simulink model "pra_tirar_print"  (R2016a)
settings: Solver=ode14x  StartTime=0.0  StopTime=30  FixedStep=0.001  RelTol=1e-3
InitFcn:
  | clear all;
  | Kpx = 10;
  | Kix = 25;
  | Kpy = 10;
  | Kiy = 25;
  | Kvphi = 3;
  | Kpphi = 2.25;
  | 
  | Kem = 0.0059;
  | Kti = 0.0059;
  | Vd = 5.4;
  | R = 1.71;
  | r = 0.072;
  | eta = 0.83;
  | N = 19;
  | 
  | Jw = 8.1e-4;
  | 
  | mi = 0.25;
  | b = .1;
  | 
  | Ts = 0.01;
  | 
  | 
  | alpha1 = 0;
  | alpha2 = 120*pi/180;
  | alpha3 = 240*pi/180;
  | g = 9.8;
  | vs = 6e-10;
  | M = 1.83;
  | l1 = 0.09;
  | l2 = 0.09;
  | l3 = 0.09;
  | r1 = 0.072;
  | r2 = 0.072;
  | r3 = 0.072;
  | kt = 0.0059;
  | kem = 0.0059;
  | N = 19;
  | L = 0.00011;
  | R = 1.71;
  | Jm1 = 3.88e-7;
  | Jm2 = 3.88e-7;
  | Jm3 = 3.88e-7;
  | J1 = 8.1e-4;
  | J2 = 8.1e-4;
  | J3 = 8.1e-4;
  | J = 2.125;
  | eta = 0.83;
  | freq = 1000; % varia entre 2.5kHz e 5Mhz
  | mic = 0.25;
  | mis = 0.25;
  | sigma0 = 100;
  | sigma1 = 0.1;
  | sigma2 = 0.1;
  | 
  | mi = 0.25;
  | b = .1;
  | 
  | kctr = kt*5.4*eta*N/(R*r1)
libraries: simulink x1
settings Model: Creator=Pichau  LastModifiedBy=Pichau

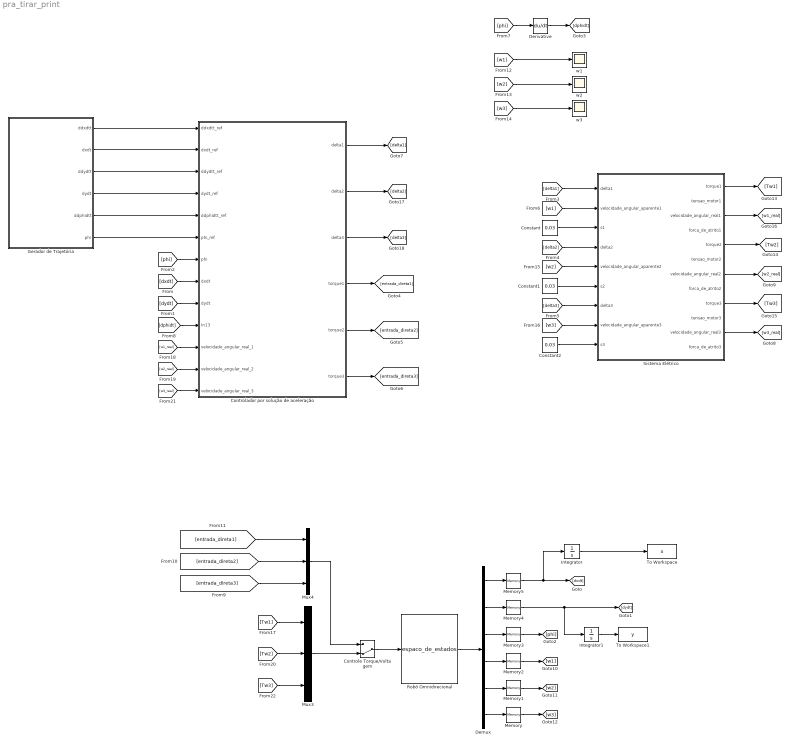
== system pra_tirar_print ==
  Constant : Constant  Value=0.03
  Constant1 : Constant  Value=0.03
  Constant2 : Constant  Value=0.03
  Controlador por solução de aceleração : Subsystem
  Controle Torque/Voltagem : ManualSwitch  CurrentSetting=0
  Demux : Demux  Outputs=6
  Derivative : Derivative
  Gerador de Trajetória : Subsystem
  Integrator : Integrator  InitialCondition=0.3
  Integrator1 : Integrator
  Memory{,1..2,4..5} (5 alike) : Memory
  Memory3 : Memory  X0=pi/2
  Mux3 : Mux  Inputs=3
  Mux4 : Mux  Inputs=3
  Robô Omnidirecional : S-Function  FunctionName=espaco_de_estados  Parameters=r,m,Jw,J,L  SFunctionDeploymentMode=off  EnableBusSupport=off  mask{r=0.072, m=1.71, Jw=8.1e-4, J=2.125, L=0.09}
      mask prompts: r "r (m)"; m "m (Kg)"; Jw "Jw (Kg*m^2)"; J "J (Kg*m^2)"; L "L (m)"
      mask Display: image(imread('Robot_omnidirectional_drive.png'));
  Sistema Elétrico : Subsystem
  To Workspace : ToWorkspace  VariableName=x  SaveFormat=Timeseries  SampleTime=-1
  To Workspace1 : ToWorkspace  VariableName=y  SaveFormat=Timeseries  SampleTime=-1
  w1 : Scope
  w2 : Scope
  w3 : Scope
  wires:
  Robô Omnidirecional/1 -> Demux/1
  Integrator1/1 -> To Workspace1/1
  Integrator/1 -> To Workspace/1
  Derivative/1 -> [dphidt]
  Mux3/1 -> Controle Torque/Voltagem/2
  Controle Torque/Voltagem/1 -> Robô Omnidirecional/1
  [w3] -> w3/1
  [w2] -> w2/1
  [w1] -> w1/1
  Demux/1 -> Memory5/1
  Demux/2 -> Memory4/1
  [phi] -> Derivative/1
  Demux/4 -> Memory2/1
  Demux/5 -> Memory1/1
  Demux/6 -> Memory/1
  Mux4/1 -> Controle Torque/Voltagem/1
  Memory/1 -> [w3]
  Memory1/1 -> [w2]
  Memory2/1 -> [w1]
  Memory4/1 -> [dydt], Integrator1/1
  Memory5/1 -> Integrator/1, [dxdt]
  Memory3/1 -> [phi]
  [entrada_direta3] -> Mux4/3
  [entrada_direta2] -> Mux4/2
  [entrada_direta1] -> Mux4/1
  Demux/3 -> Memory3/1
  Sistema Elétrico/5(torque2) -> [Tw2]
  Sistema Elétrico/9(torque3) -> [Tw3]
  Sistema Elétrico/1(torque1) -> [Tw1]
  [w1] -> Sistema Elétrico/2(velocidade_angular_aparente1)
  [delta2] -> Sistema Elétrico/4(delta2)
  [w2] -> Sistema Elétrico/5(velocidade_angular_aparente2)
  [delta3] -> Sistema Elétrico/7(delta3)
  [w3] -> Sistema Elétrico/8(velocidade_angular_aparente3)
  Sistema Elétrico/3(velocidade_angular_real1) -> [w1_real]
  Sistema Elétrico/7(velocidade_angular_real2) -> [w2_real]
  Sistema Elétrico/11(velocidade_angular_real3) -> [w3_real]
  [Tw1] -> Mux3/1
  [Tw2] -> Mux3/2
  [Tw3] -> Mux3/3
  Gerador de Trajetória/1(ddxdtt) -> Controlador por solução de aceleração/1(ddxdtt_ref)
  Gerador de Trajetória/2(dxdt) -> Controlador por solução de aceleração/2(dxdt_ref)
  Gerador de Trajetória/3(ddydtt) -> Controlador por solução de aceleração/3(ddydtt_ref)
  Gerador de Trajetória/4(dydt) -> Controlador por solução de aceleração/4(dydt_ref)
  Gerador de Trajetória/5("ddphidtt ") -> Controlador por solução de aceleração/5(ddphidtt_ref)
  Gerador de Trajetória/6(phi) -> Controlador por solução de aceleração/6(phi_ref)
  [phi] -> Controlador por solução de aceleração/7(phi)
  [dxdt] -> Controlador por solução de aceleração/8(dxdt)
  [dydt] -> Controlador por solução de aceleração/9(dydt)
  [dphidt] -> Controlador por solução de aceleração/10(In13)
  [w2_real] -> Controlador por solução de aceleração/12(velocidade_angular_real_2)
  [w3_real] -> Controlador por solução de aceleração/13(velocidade_angular_real_3)
  [w1_real] -> Controlador por solução de aceleração/11(velocidade_angular_real_1)
  Controlador por solução de aceleração/5(torque2) -> [entrada_direta2]
  Controlador por solução de aceleração/6(torque3) -> [entrada_direta3]
  Controlador por solução de aceleração/4(torque1) -> [entrada_direta1]
  Controlador por solução de aceleração/1(delta1) -> [delta1]
  Controlador por solução de aceleração/2(delta2) -> [delta2]
  Controlador por solução de aceleração/3(delta3) -> [delta3]
  [delta1] -> Sistema Elétrico/1(delta1)
  Constant/1 -> Sistema Elétrico/3(s1)
  Constant1/1 -> Sistema Elétrico/6(s2)
  Constant2/1 -> Sistema Elétrico/9(s3)

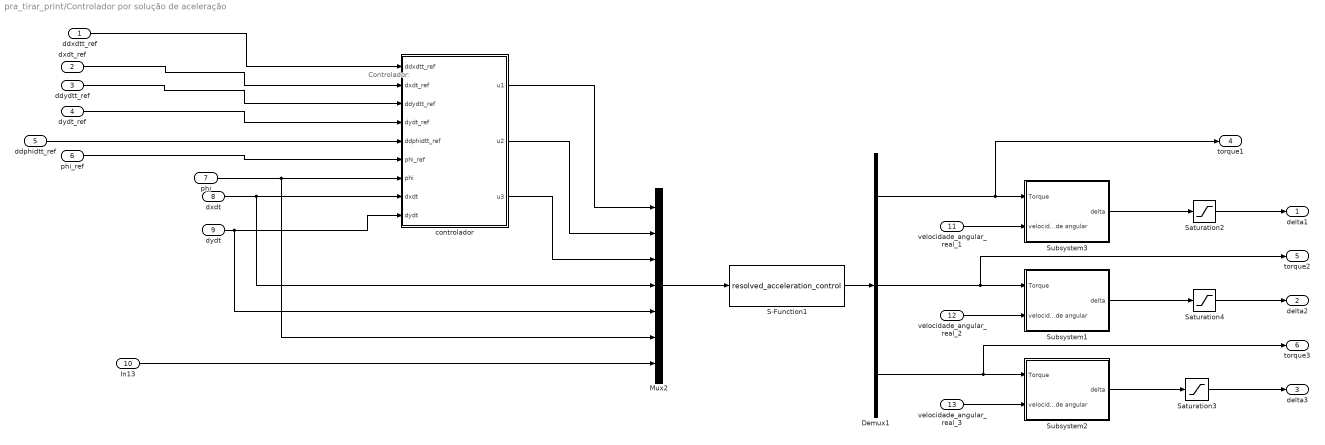
== system pra_tirar_print/Controlador por solução de aceleração ==
  note: Controlador:
  ddxdtt_ref : Inport
  dxdt_ref : Inport  Port=2
  ddydtt_ref : Inport  Port=3
  dydt_ref : Inport  Port=4
  ddphidtt_ref : Inport  Port=5
  phi_ref : Inport  Port=6
  phi : Inport  Port=7
  dxdt : Inport  Port=8
  dydt : Inport  Port=9
  In13 : Inport  Port=10
  velocidade_angular_real_1 : Inport  Port=11
  velocidade_angular_real_2 : Inport  Port=12
  velocidade_angular_real_3 : Inport  Port=13
  Demux1 : Demux  Outputs=3
  Mux2 : Mux  Inputs=7
  S-Function1 : S-Function  FunctionName=resolved_acceleration_control  Parameters=r,L,m,J,Jw  SFunctionDeploymentMode=off  EnableBusSupport=off  mask{r=0.072, L=0.09, m=1.71, J=2.125, Jw=8.1e-4}
  Saturation2 : Saturate  UpperLimit=1  LowerLimit=-1
  Saturation3 : Saturate  UpperLimit=1  LowerLimit=-1
  Saturation4 : Saturate  UpperLimit=1  LowerLimit=-1
  Subsystem1 : Subsystem
  Subsystem2 : Subsystem
  Subsystem3 : Subsystem
  controlador : Subsystem
  delta1 : Outport
  delta2 : Outport  Port=2
  delta3 : Outport  Port=3
  torque1 : Outport  Port=4
  torque2 : Outport  Port=5
  torque3 : Outport  Port=6
  wires:
  controlador/1(u1) -> Mux2/1
  controlador/3(u3) -> Mux2/3
  controlador/2(u2) -> Mux2/2
  Demux1/3 -> torque3/1, Subsystem2/1(Torque)
  ddxdtt_ref/1 -> controlador/1(ddxdtt_ref)
  dydt_ref/1 -> controlador/4(dydt_ref)
  ddydtt_ref/1 -> controlador/3(ddydtt_ref)
  dxdt_ref/1 -> controlador/2(dxdt_ref)
  phi/1 -> Mux2/6, controlador/7(phi)
  S-Function1/1 -> Demux1/1
  ddphidtt_ref/1 -> controlador/5(ddphidtt_ref)
  dxdt/1 -> Mux2/4, controlador/8(dxdt)
  dydt/1 -> Mux2/5, controlador/9(dydt)
  phi_ref/1 -> controlador/6(phi_ref)
  Mux2/1 -> S-Function1/1
  velocidade_angular_real_3/1 -> Subsystem2/2(velocidade angular)
  Subsystem2/1(delta) -> Saturation3/1
  velocidade_angular_real_1/1 -> Subsystem3/2(velocidade angular)
  Subsystem3/1(delta) -> Saturation2/1
  velocidade_angular_real_2/1 -> Subsystem1/2(velocidade angular)
  Demux1/1 -> torque1/1, Subsystem3/1(Torque)
  Subsystem1/1(delta) -> Saturation4/1
  In13/1 -> Mux2/7
  Saturation2/1 -> delta1/1
  Demux1/2 -> torque2/1, Subsystem1/1(Torque)
  Saturation3/1 -> delta3/1
  Saturation4/1 -> delta2/1

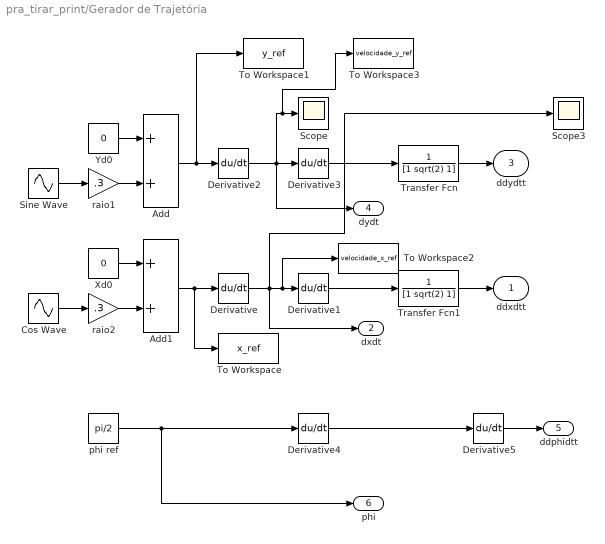
== system pra_tirar_print/Gerador de Trajetória ==
  Add : Sum
  Add1 : Sum
  Cos Wave : Sin  Frequency=0.3  Phase=pi/2  SampleTime=0
  Derivative{,1..5} (6 alike) : Derivative
  Scope : Scope
  Scope3 : Scope
  Sine Wave : Sin  Frequency=0.3  SampleTime=0
  To Workspace : ToWorkspace  VariableName=x_ref  SaveFormat=Timeseries  SampleTime=-1
  To Workspace1 : ToWorkspace  VariableName=y_ref  SaveFormat=Timeseries  SampleTime=-1
  To Workspace2 : ToWorkspace  VariableName=velocidade_x_ref  SaveFormat=Timeseries  SampleTime=-1
  To Workspace3 : ToWorkspace  VariableName=velocidade_y_ref  SaveFormat=Timeseries  SampleTime=-1
  Transfer Fcn : TransferFcn  Denominator=[1 sqrt(2) 1]
  Transfer Fcn1 : TransferFcn  Denominator=[1 sqrt(2) 1]
  Xd0 : Constant  Value=0
  Yd0 : Constant  Value=0
  phi ref : Constant  Value=pi/2
  raio1 : Gain  Gain=.3
  raio2 : Gain  Gain=.3
  ddxdtt : Outport
  dxdt : Outport  Port=2
  ddydtt : Outport  Port=3
  dydt : Outport  Port=4
  "ddphidtt " : Outport  Port=5
  phi : Outport  Port=6
  wires:
  Transfer Fcn1/1 -> ddxdtt/1
  Transfer Fcn/1 -> ddydtt/1
  Derivative1/1 -> Transfer Fcn1/1
  Derivative3/1 -> Transfer Fcn/1
  Derivative2/1 -> Derivative3/1, To Workspace3/1, Scope/1, dydt/1
  Derivative/1 -> Scope3/1, To Workspace2/1, Derivative1/1, dxdt/1
  Sine Wave/1 -> raio1/1
  raio1/1 -> Add/2
  Add/1 -> To Workspace1/1, Derivative2/1
  Add1/1 -> To Workspace/1, Derivative/1
  raio2/1 -> Add1/2
  Cos Wave/1 -> raio2/1
  Xd0/1 -> Add1/1
  Yd0/1 -> Add/1
  phi ref/1 -> Derivative4/1, phi/1
  Derivative4/1 -> Derivative5/1
  Derivative5/1 -> "ddphidtt "/1

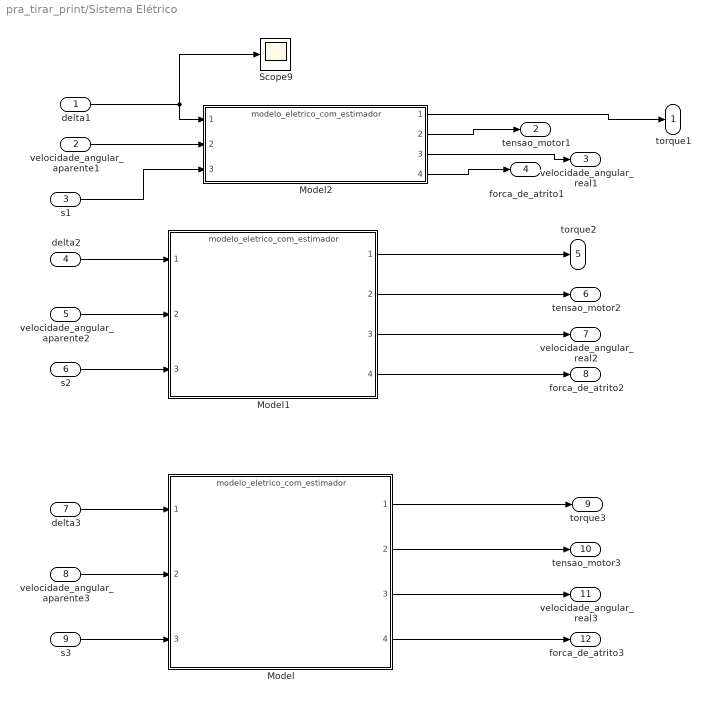
== system pra_tirar_print/Sistema Elétrico ==
  delta1 : Inport
  velocidade_angular_aparente1 : Inport  Port=2
  s1 : Inport  Port=3
  delta2 : Inport  Port=4
  velocidade_angular_aparente2 : Inport  Port=5
  s2 : Inport  Port=6
  delta3 : Inport  Port=7
  velocidade_angular_aparente3 : Inport  Port=8
  s3 : Inport  Port=9
  Model : ModelReference  ModelNameDialog=modelo_eletrico_com_estimador  SimulationMode=Normal  ModelReferenceVersion=1.41
  Model1 : ModelReference  ModelNameDialog=modelo_eletrico_com_estimador  SimulationMode=Normal  ModelReferenceVersion=1.41
  Model2 : ModelReference  ModelNameDialog=modelo_eletrico_com_estimador  SimulationMode=Normal  ModelReferenceVersion=1.41
  Scope9 : Scope
  torque1 : Outport
  tensao_motor1 : Outport  Port=2
  velocidade_angular_real1 : Outport  Port=3
  forca_de_atrito1 : Outport  Port=4
  torque2 : Outport  Port=5
  tensao_motor2 : Outport  Port=6
  velocidade_angular_real2 : Outport  Port=7
  forca_de_atrito2 : Outport  Port=8
  torque3 : Outport  Port=9
  tensao_motor3 : Outport  Port=10
  velocidade_angular_real3 : Outport  Port=11
  forca_de_atrito3 : Outport  Port=12
  wires:
  delta3/1 -> Model/1
  velocidade_angular_aparente1/1 -> Model2/2
  Model/2 -> tensao_motor3/1
  velocidade_angular_aparente2/1 -> Model1/2
  delta1/1 -> Scope9/1, Model2/1
  Model2/2 -> tensao_motor1/1
  Model1/2 -> tensao_motor2/1
  delta2/1 -> Model1/1
  velocidade_angular_aparente3/1 -> Model/2
  Model1/3 -> velocidade_angular_real2/1
  Model2/4 -> forca_de_atrito1/1
  Model1/4 -> forca_de_atrito2/1
  Model/3 -> velocidade_angular_real3/1
  Model/4 -> forca_de_atrito3/1
  Model2/3 -> velocidade_angular_real1/1
  Model/1 -> torque3/1
  Model2/1 -> torque1/1
  Model1/1 -> torque2/1
  s1/1 -> Model2/3
  s2/1 -> Model1/3
  s3/1 -> Model/3

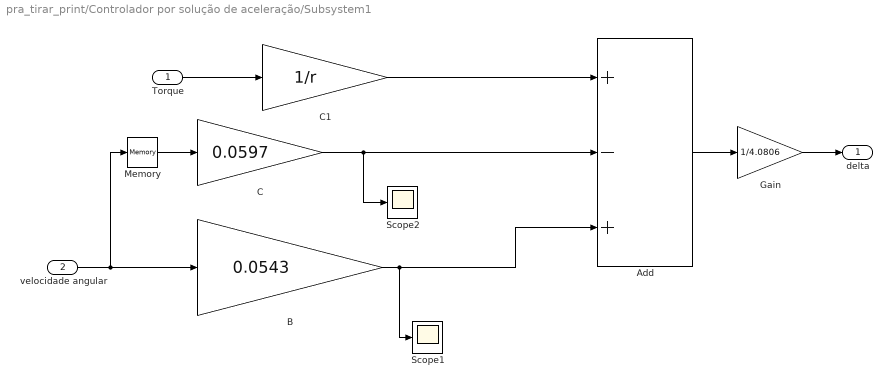
== system pra_tirar_print/Controlador por solução de aceleração/Subsystem1 ==
  Torque : Inport
  velocidade angular : Inport  Port=2
  Add : Sum  Inputs=+-+
  B : Gain  Gain=0.0543
  C : Gain  Gain=0.0597
  C1 : Gain  Gain=1/r
  Gain : Gain  Gain=1/4.0806
  Memory : Memory
  Scope1 : Scope
  Scope2 : Scope
  delta : Outport
  wires:
  C1/1 -> Add/1
  Add/1 -> Gain/1
  velocidade angular/1 -> Memory/1, B/1
  Torque/1 -> C1/1
  Memory/1 -> C/1
  Gain/1 -> delta/1
  C/1 -> Scope2/1, Add/2
  B/1 -> Scope1/1, Add/3

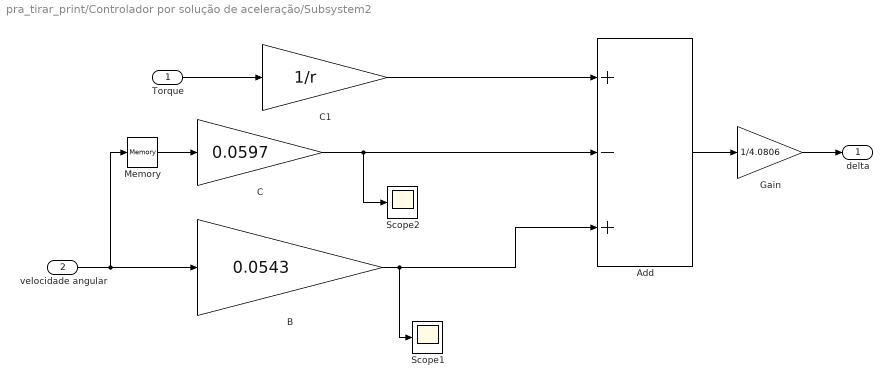
== system pra_tirar_print/Controlador por solução de aceleração/Subsystem2 ==
  Torque : Inport
  velocidade angular : Inport  Port=2
  Add : Sum  Inputs=+-+
  B : Gain  Gain=0.0543
  C : Gain  Gain=0.0597
  C1 : Gain  Gain=1/r
  Gain : Gain  Gain=1/4.0806
  Memory : Memory
  Scope1 : Scope
  Scope2 : Scope
  delta : Outport
  wires:
  B/1 -> Add/3, Scope1/1
  C/1 -> Add/2, Scope2/1
  Gain/1 -> delta/1
  Memory/1 -> C/1
  Torque/1 -> C1/1
  velocidade angular/1 -> B/1, Memory/1
  Add/1 -> Gain/1
  C1/1 -> Add/1

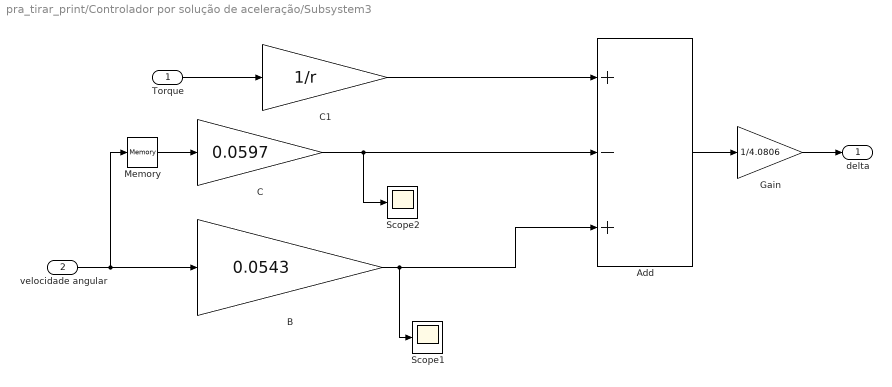
== system pra_tirar_print/Controlador por solução de aceleração/Subsystem3 ==
  Torque : Inport
  velocidade angular : Inport  Port=2
  Add : Sum  Inputs=+-+
  B : Gain  Gain=0.0543
  C : Gain  Gain=0.0597
  C1 : Gain  Gain=1/r
  Gain : Gain  Gain=1/4.0806
  Memory : Memory
  Scope1 : Scope
  Scope2 : Scope
  delta : Outport
  wires:
  B/1 -> Add/3, Scope1/1
  C/1 -> Add/2, Scope2/1
  Gain/1 -> delta/1
  Memory/1 -> C/1
  Torque/1 -> C1/1
  velocidade angular/1 -> B/1, Memory/1
  Add/1 -> Gain/1
  C1/1 -> Add/1

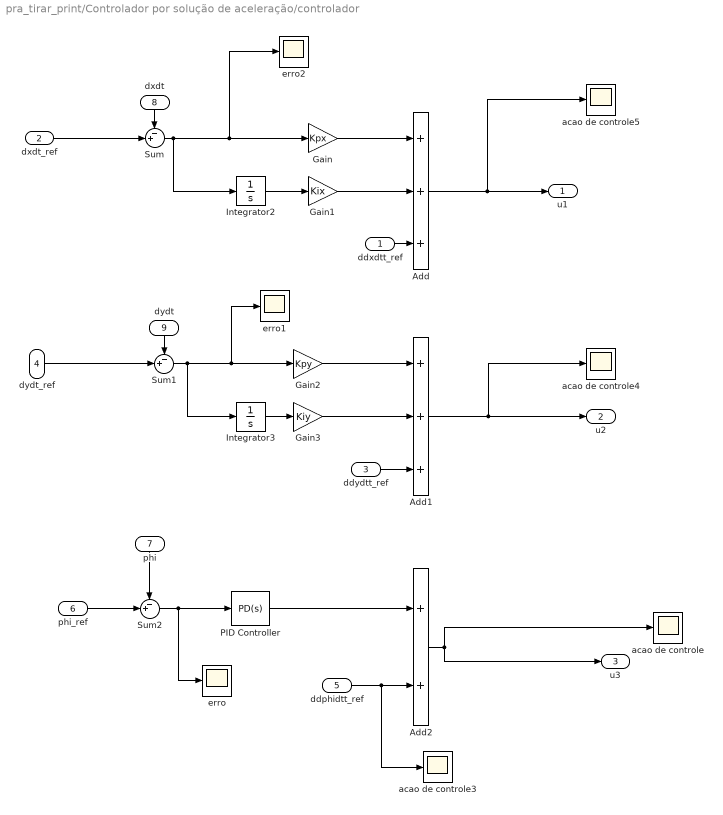
== system pra_tirar_print/Controlador por solução de aceleração/controlador ==
  ddxdtt_ref : Inport
  dxdt_ref : Inport  Port=2
  ddydtt_ref : Inport  Port=3
  dydt_ref : Inport  Port=4
  ddphidtt_ref : Inport  Port=5
  phi_ref : Inport  Port=6
  phi : Inport  Port=7
  dxdt : Inport  Port=8
  dydt : Inport  Port=9
  Add : Sum  Inputs=+++
  Add1 : Sum  Inputs=+++
  Add2 : Sum
  Gain : Gain  Gain=Kpx
  Gain1 : Gain  Gain=Kix
  Gain2 : Gain  Gain=Kpy
  Gain3 : Gain  Gain=Kiy
  Integrator2 : Integrator
  Integrator3 : Integrator
  PID Controller : simulink/Continuous/PID Controller  Controller=PD  TimeDomain=Continuous-time  SampleTime=-1  IntegratorMethod=Forward Euler  FilterMethod=Forward Euler  Form=Parallel  UseFilter=on  ControllerParametersSource=internal  P=2.25  I=0  D=3  N=100  InitialConditionSource=internal  InitialConditionForIntegrator=0  InitialConditionForFilter=0  ExternalReset=none  LimitOutput=off  UpperSaturationLimit=inf  LowerSaturationLimit=-inf  LinearizeAsGain=on  AntiWindupMode=none  Kb=1  TrackingMode=off  Kt=1  PParamMin=[]  PParamMax=[]  IParamMin=[]  IParamMax=[]  DParamMin=[]  DParamMax=[]  NParamMin=[]  NParamMax=[]  KbParamMin=[]  KbParamMax=[]  KtParamMin=[]  KtParamMax=[]  POutMin=[]  POutMax=[]  IOutMin=[]  IOutMax=[]  DOutMin=[]  DOutMax=[]  NOutMin=[]  NOutMax=[]  KbOutMin=[]  KbOutMax=[]  KtOutMin=[]  KtOutMax=[]  IntegratorOutMin=[]  IntegratorOutMax=[]  FilterOutMin=[]  FilterOutMax=[]  SumOutMin=[]  SumOutMax=[]  SumI1OutMin=[]  SumI1OutMax=[]  SumI2OutMin=[]  SumI2OutMax=[]  SumI3OutMin=[]  SumI3OutMax=[]  SumDOutMin=[]  SumDOutMax=[]  SaturationOutMin=[]  SaturationOutMax=[]  IntegratorContinuousStateAttributes=''  IntegratorStateMustResolveToSignalObject=off  IntegratorRTWStateStorageClass=Auto  FilterContinuousStateAttributes=''  FilterStateMustResolveToSignalObject=off  FilterRTWStateStorageClass=Auto  DifferentiatorICPrevScaledInput=0  DifferentiatorOutMin=[]  DifferentiatorOutMax=[]
  Sum : Sum  Inputs=-+|
  Sum1 : Sum  Inputs=-+|
  Sum2 : Sum  Inputs=-+|
  acao de controle{,3..5} (4 alike) : Scope
  erro : Scope
  erro1 : Scope
  erro2 : Scope
  u1 : Outport
  u2 : Outport  Port=2
  u3 : Outport  Port=3
  wires:
  Sum2/1 -> erro/1, PID Controller/1
  Sum1/1 -> erro1/1, Gain2/1, Integrator3/1
  Gain1/1 -> Add/2
  Integrator2/1 -> Gain1/1
  dydt_ref/1 -> Sum1/2
  Gain2/1 -> Add1/1
  Integrator3/1 -> Gain3/1
  Sum/1 -> erro2/1, Gain/1, Integrator2/1
  Gain3/1 -> Add1/2
  ddphidtt_ref/1 -> acao de controle3/1, Add2/2
  ddydtt_ref/1 -> Add1/3
  ddxdtt_ref/1 -> Add/3
  phi/1 -> Sum2/1
  dxdt_ref/1 -> Sum/2
  dxdt/1 -> Sum/1
  phi_ref/1 -> Sum2/2
  Gain/1 -> Add/1
  dydt/1 -> Sum1/1
  Add1/1 -> acao de controle4/1, u2/1
  Add/1 -> acao de controle5/1, u1/1
  Add2/1 -> u3/1, acao de controle/1
  PID Controller/1 -> Add2/1
